simulink model "LSAS"  (Simulink 7.5)
settings: Solver=ode45  StartTime=0.0  StopTime=20.0  RelTol=1e-3
settings Model: Creator=Drew Gross  LastModifiedBy=Jake

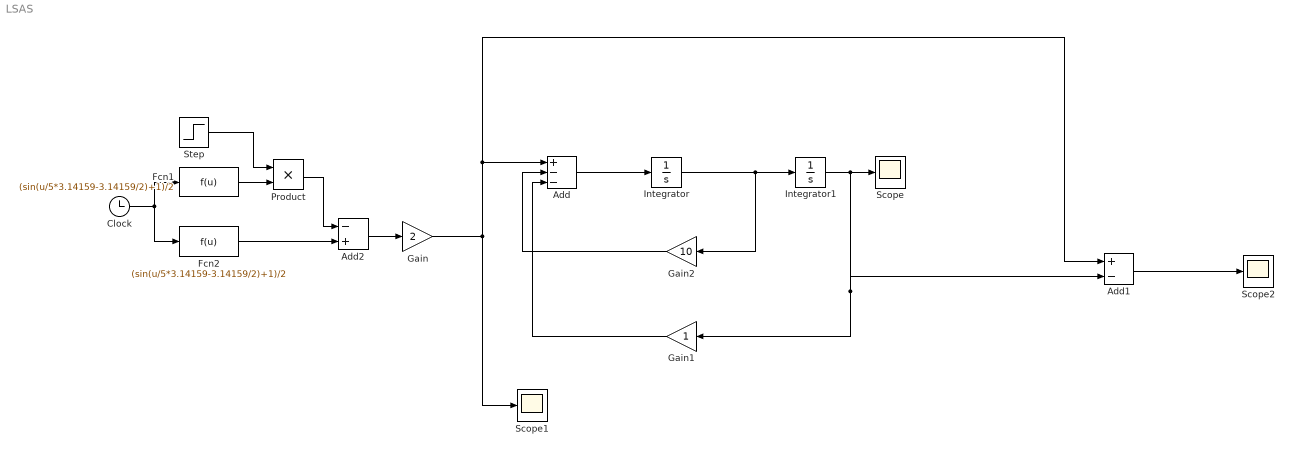
== system LSAS ==
  Add : Sum  Inputs=+--  OutDataType=fixdt(1, 16)  OutScaling=2^-10
  Add1 : Sum  Inputs=+-  OutDataType=fixdt(1, 16)  OutScaling=2^-10
  Add2 : Sum  Inputs=-+  OutDataType=fixdt(1, 16)  OutScaling=2^-10
  Clock : Clock
  Fcn1 : Fcn  Expr=(sin(u/5*3.14159-3.14159/2)+1)/2
  Fcn2 : Fcn  Expr=(sin(u/5*3.14159-3.14159/2)+1)/2
  Gain : Gain  Gain=2  ParameterDataType=fixdt(1, 16)  ParameterScaling=2^0  OutDataType=fixdt(1, 16)  OutScaling=2^0
  Gain1 : Gain  ParameterDataType=fixdt(1, 16)  ParameterScaling=2^0  OutDataType=fixdt(1, 16)  OutScaling=2^0
  Gain2 : Gain  Gain=10  ParameterDataType=fixdt(1, 16)  ParameterScaling=2^0  OutDataType=fixdt(1, 16)  OutScaling=2^0
  Integrator : Integrator
  Integrator1 : Integrator
  Product : Product  OutDataType=fixdt(1, 16)  OutScaling=2^0  RndMeth=Zero
  Scope : Scope
      settings: TimeRange=20
  Scope1 : Scope
  Scope2 : Scope
      settings: SaveName=ScopeData2
  Step : Step  Time=10  SampleTime=0
  wires:
  Integrator/1 -> Integrator1/1, Gain2/1
  Integrator1/1 -> Scope/1, Gain1/1, Add1/2
  Add/1 -> Integrator/1
  Gain2/1 -> Add/2
  Gain1/1 -> Add/3
  Add1/1 -> Scope2/1
  Clock/1 -> Fcn1/1, Fcn2/1
  Fcn1/1 -> Product/2
  Step/1 -> Product/1
  Product/1 -> Add2/1
  Fcn2/1 -> Add2/2
  Add2/1 -> Gain/1
  Gain/1 -> Scope1/1, Add/1, Add1/1
